simulink model "FCS"  (R2020b)
settings: Solver=VariableStepAuto  StartTime=0.0  StopTime=stabtime+twdw  RelTol=1e-3
undefined symbols (not defined in the file): Capacity, CombinedEDMElectricalPower, CombinedEDMLoss, fuelCellOrg, N, Nom_voltage, OPCircuitDechg, Rincharge, RInDechrg, sigbuilder_block, SOC_initial, SOCR, Time
libraries: powerlib_meascontrol x6, eeStairGenerator x5, simulink x2, powerlib x1
settings Model: Creator=oqz0vm8  LastModifiedBy=dahmani
settings SolverCC: AlgebraicLoopSolver=LineSearch
settings DataIOCC: ReturnWorkspaceOutputs=off
settings DebuggingCC: ArithmeticOperatorsInVariantConditions=warning
settings SFSimCC: SimUseLocalCustomCode=off  CustomCodeUndefinedFunction=UseInterfaceOnly
settings RTWCC: RTWUseLocalCustomCode=off
settings CodeAppCC: StateflowObjectComments=on
settings SimscapeCC: SimscapeNormalizeSystem=off

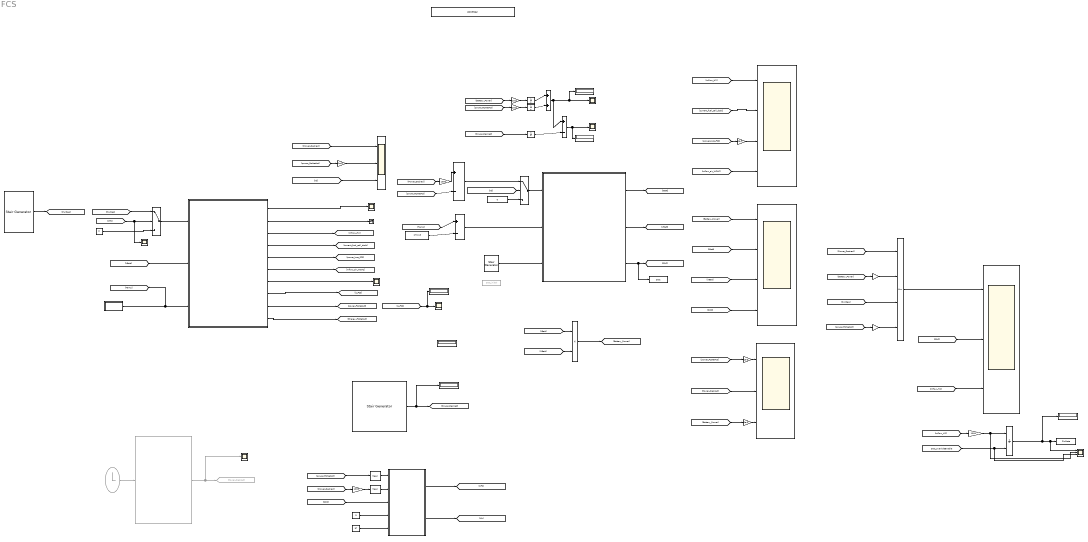
== system FCS ==
  note: Energy balance
  "  " : Gain  Gain=1e-3
  Battery_Model1 : Subsystem
  Clock : Clock  Commented=on
  Combined Drive Motor : Subsystem  Commented=on
  Constant : Constant  Value=273.15
  Constant1 : Constant  Value=0
  Constant4 : Constant  Value=0
  Display{,1..4,6} (6 alike) : Display
  EMS : MATLAB Function  TreatAsAtomicUnit=on
  Gain1 : Gain  Gain=1000
  Gain2 : Gain  Gain=1e-3
  Gain3 : Gain  Gain=1e-3
  Gain4 : Gain  Gain=1000
  Goto : Goto  Commented=on  GotoTag=Power_Desired
  Integrator : Integrator
  Integrator1 : Integrator
  Integrator2 : Integrator
  Integrator3 : Integrator  ExternalReset=either
  "K to °C " : Sum  Inputs=|+-
  "KW to W " : Gain  Gain=1000
  Mean : powerlib_meascontrol/Measurements/Mean  Freq=60  Vinit=1  Ts=0
  Mean1 : powerlib_meascontrol/Measurements/Mean  Freq=60  Vinit=1  Ts=0
  Mux : Mux
  Product : Product
  SOC_initial : eeStairGenerator/Stair Generator  LabelModeActiveChoice=Discrete  TimeInput=SOCInitTime  AmplitudeInput=SOC_overrideValue  SampleTime=1  RepeatPattern=off  OutDataTypeStr=double
      settings: SourceProductBaseCode=PS
  SOC_initial1 : Constant  Commented=on  Value=SOC_initial
  SOCmax : Constant  Value=97
  SOCmin : Constant  Value=3
  Scope : Scope  NumInputPorts=4
  Scope{1..2,5..6,9..10,14} (7 alike) : Scope
  Scope{7..8,11..12} (4 alike) : Scope  NumInputPorts=3
  Scope4 : Scope  NumInputPorts=4
  Stair Generator : eeStairGenerator/Stair Generator  LabelModeActiveChoice=Discrete  TimeInput=FCSimPdesTime  AmplitudeInput=FCSimPdes  SampleTime=1  RepeatPattern=off  OutDataTypeStr=double
      settings: SourceProductBaseCode=PS
  Stair Generator1 : eeStairGenerator/Stair Generator  LabelModeActiveChoice=Discrete  TimeInput=PwrReqTime  AmplitudeInput=PwrReq  SampleTime=1  RepeatPattern=off  OutDataTypeStr=double
      settings: SourceProductBaseCode=PS
  Sum : Sum  Inputs=|+-
  Sum1 : Sum  Inputs=|++
  Sum2 : Sum  Inputs=|+-
  Switch1 : Switch  Criteria=u2 > Threshold
  Switch3 : Switch  Criteria=u2 > Threshold
  Temp(K) : Subsystem  Tag=STV Subsys  LoadFcn=sigbuilder_block('load');  StartFcn=sigbuilder_block('start');  StopFcn=sigbuilder_block('stop');  ClipboardFcn=sigbuilder_block('clipboard');  mask(Sigbuilder block){tuvar=[0:10]}
      mask help: Simulink:masks:SigbuilderBlock_MD
      mask init:
      | if ~strcmp(get_param(bdroot(gcbh),'SimulationStatus'),'stopped') tuvar = sigbuilder_block('maskInit'); end
      settings: CopyFcn=sigbuilder_block('copy');  DeleteFcn=sigbuilder_block('delete');  ModelCloseFcn=sigbuilder_block('modelClose');  PreSaveFcn=sigbuilder_block('preSave');  PauseFcn=sigbuilder_block('pause');  ContinueFcn=sigbuilder_block('continue');  NameChangeFcn=sigbuilder_block('namechange');  OpenFcn=sigbuilder_block('open',[595.8 21.6 550.8 361.2 ]);  CloseFcn=sigbuilder_block('close');
      mask Display: plot(0, 0, 100, 100,[2, 2, 32, 32, 2], [68, 8, 8, 68, 68],[32, 2], [38, 38], [32, 19, 2],[53, 60, 44], [32, 17, 17, 2],[16, 16, 31, 31]);txt = getActiveGroup(gcbh);text(2, 100, txt,'verticalAlignment', 'top');
  Terminator : Terminator
  To Workspace : ToWorkspace  VariableName=FlwRate  SampleTime=-1
      settings: Save2DSignal=2-D array (concatenate along first dimension)
  To Workspace2 : ToWorkspace  VariableName=SOC  SaveFormat=Timeseries  SampleTime=-1
      settings: Save2DSignal=2-D array (concatenate along first dimension)
  W to KW : Gain  Gain=1e-3
  W to KW {1..4} (4 alike) : Gain  Gain=1e-3
  fuelCell_DCDC_Boost_Models : Subsystem
  powergui : powerlib/powergui  Priority=1  SimulationMode=Continuous  SampleTime=50e-6  frequency=60  Iterations=50  frequencyindice=0  Pbase=100e6  ErrMax=1e-4  UnitsV=kV  UnitsW=MW  buscounter=0  FunctionMessages=off  echomessages=off  EnableUseOfTLC=off  CurrentSourceSwitches=off  DisableSnubberDevices=off  DisableRonSwitches=off  DisableVfSwitches=off  DisplayEquations=off  AutomaticDiscreteSolvers=off  SolverType=Tustin/Backward Euler (TBE)  Interpol=off  ExternalGateDelay=off  methode=off  Ts=100  x0status=blocks  SPID=on  SwTol=0  HookPort=off  NonlinearTolerance=1e-4  nMaxIteration=100  ContinueOnMaxIteration=off  RestoreLinks=warning  ResistiveCurrentMeasurement=off  Frange=[0:2:500]  Ylog=off  Xlog=on  ShowGrid=off  save=off  variable=ZData  structure=0  ZoomFFT=off  StartTime=0.0  cycles=1  DisplayStyle=1  fundamental=60  FreqAxis=off  MaxFrequency=1000  frequencyindicesteady=1  RmsSteady=1  display=off
  wires:
  [SOC] -> EMS/3(SOC)
  [Battery_Power] -> Scope/1  "Battery_Power"
  W to KW 4/1 -> Scope4/3  "power_loss_FCS"
  [Kb] -> Switch3/2
  EMS/1(KFC) -> [KFC]
  SOCmin/1 -> EMS/4(SOCmin)
  Temp(K)/1(Signal 1) -> [Temp], fuelCell_DCDC_Boost_Models/3(temp_air_atmo_[K])
  Mean1/1 -> EMS/2(PL)
  Combined Drive Motor/1(Power_Desired_net(KW)) -> Scope2/1, Goto/1
  [Kb] -> Scope8/3
  "KW to W "/1 -> Sum/1
  [VBatt] -> Product/2
  fuelCell_DCDC_Boost_Models/5(power_loss_FCS_[W]) -> [power_loss_FCS]
  [power_loss_FCS] -> W to KW 4/1
  [power_FcsNetAct] -> W to KW 3/1
  Sum/1 -> Switch3/1
  Switch3/1 -> Battery_Model1/1(P_demand(w))
  [power_FcsNetAct] -> Sum/2
  fuelCell_DCDC_Boost_Models/9(power_FcsNetAct) -> [power_FcsNetAct]
  "K to °C "/1 -> Battery_Model1/2(Temp(Cels))
  [Battery_Power] -> W to KW 1/1
  W to KW 3/1 -> Scope8/2  "FuelCell_Power"
  Constant4/1 -> Switch3/3
  [Power_Desired] -> "KW to W "/1
  W to KW 2/1 -> Scope7/1  "FuelCell_Power"
  [Power_Desired] -> Gain1/1
  [Power_Desired] -> Scope7/2  "Power_Desired"
  SOCmax/1 -> EMS/5(SOCmax)
  [Power_Desired] -> Scope8/1  "Power_Desired"
  [mflow_air_WCAC] -> Scope4/4  "mflow_air_WCAC"
  fuelCell_DCDC_Boost_Models/1(info) -> Scope1/1
  fuelCell_DCDC_Boost_Models/2(sensor) -> Terminator/1
  [current_fuel_cell_dcdc] -> Scope4/2  "current_fuel_cell_dcdc"
  [power_FcsNetAct] -> W to KW 2/1
  [mflow_H2] -> Scope4/1  "mflow_H2"
  W to KW 1/1 -> Scope7/3  "Battery_Power"
  EMS/2(Kb) -> [Kb]
  fuelCell_DCDC_Boost_Models/8(U_FCS[V]) -> [U_FCS]
  Gain1/1 -> Mean1/1
  [SOC] -> Scope/4  "SOC"
  [power_FcsNetAct] -> Mean/1
  fuelCell_DCDC_Boost_Models/4(current_fuel_cell_dcdc_[A]) -> [current_fuel_cell_dcdc]
  Mean/1 -> EMS/1(PFC)
  fuelCell_DCDC_Boost_Models/6(mflow_air_WCAC_[kg.s-1]) -> [mflow_air_WCAC]
  [IBatt] -> Product/1
  [IBatt] -> Scope/2  "Battery_current"
  Battery_Model1/3(.SOC) -> To Workspace2/1, [SOC]
  Clock/1 -> Combined Drive Motor/1(Time(s))
  [U_FCS] -> Display2/1, Scope5/1
  Constant/1 -> "K to °C "/2
  Battery_Model1/2(.VBatt) -> [VBatt]
  [VBatt] -> Scope/3  "Battery_voltage"
  Battery_Model1/1(Ibat) -> [IBatt]
  fuelCell_DCDC_Boost_Models/7(power_StackAct_[W]) -> Scope6/1
  [Temp] -> "K to °C "/1
  Sum2/1 -> Scope10/1, Display/1
  Sum1/1 -> Display1/1, Scope14/1, Sum2/1
  [Battery_Power] -> "  "/1
  Integrator/1 -> Sum1/2
  Integrator2/1 -> Sum2/2
  W to KW/1 -> Integrator/1
  Integrator1/1 -> Sum1/1
  [power_FcsNetAct] -> W to KW/1
  [Power_Desired] -> Integrator2/1
  "  "/1 -> Integrator1/1
  [VBatt] -> fuelCell_DCDC_Boost_Models/2(voltage_out_epsBattTracOrg_[V])
  SOC_initial/1 -> Battery_Model1/3(SOC_initial)
  Stair Generator/1 -> Display4/1, [Power_Desired]
  fuelCell_DCDC_Boost_Models/3(mflow_H2_[kg.s-1]) -> [mflow_H2]
  Constant1/1 -> Switch1/3
  [PwrReq] -> Switch1/1
  [KFC] -> Scope9/1, Switch1/2
  Switch1/1 -> fuelCell_DCDC_Boost_Models/1(FcsPwrReq(Kw))
  Stair Generator1/1 -> [PwrReq]
  [Power_Desired] -> Mux/1  "Power_Desired"
  Mux/1 -> Scope12/1
  [Battery_Power] -> Gain2/1
  Gain2/1 -> Mux/2  "Battery_Power"
  [PwrReq] -> Mux/3  "PwrReq"
  [power_FcsNetAct] -> Gain3/1
  Gain3/1 -> Mux/4  "power_FcsNetAct"
  [SOC] -> Scope12/2  "SOC"
  [mflow_H2] -> Scope12/3  "mflow_H2"
  [SOC_overrideEnable] -> Scope11/3, Integrator3/2  "SOC_overrideEnable"
  Integrator3/1 -> Display6/1, Scope11/1, To Workspace/1
  [mflow_H2] -> Gain4/1
  Gain4/1 -> Scope11/2, Integrator3/1
  fuelCell_DCDC_Boost_Models/10(Energy_FcsNetAct) -> [Energy_FcsNetAct]
  Product/1 -> [Battery_Power]

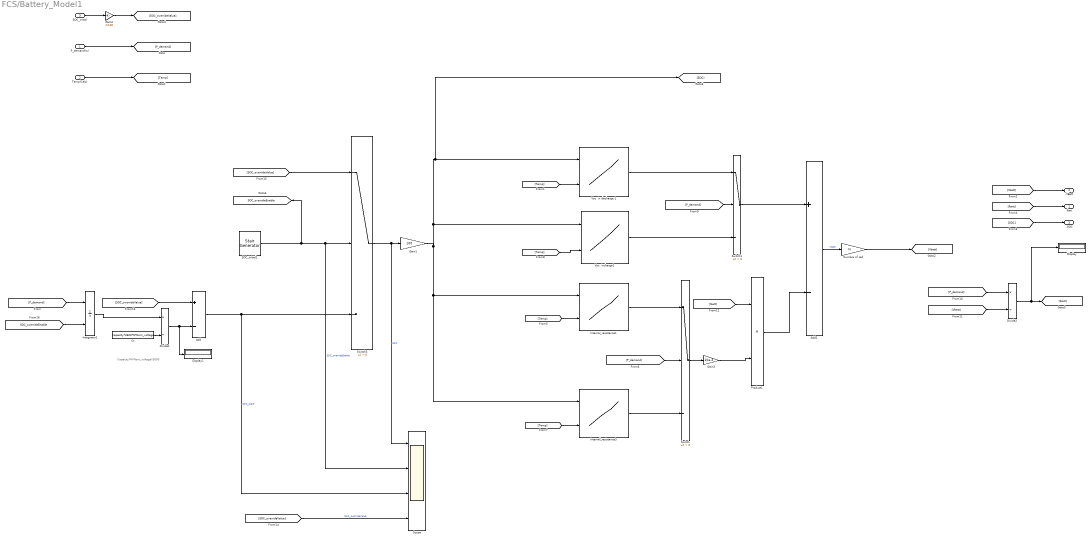
== system FCS/Battery_Model1 ==
  note: Capacity*N*Nom_voltage*3600
  P_demand(w) : Inport
  Temp(Cels) : Inport  Port=2
  SOC_initial : Inport  Port=3
  Add : Sum  Inputs=+-
  Add2 : Sum  Inputs=+-
  "Ct " : Constant  Value=Capacity*3600*N*Nom_voltage
  Display : Display
  Display1 : Display
  Divide1 : Product  Inputs=*/
  Divide2 : Product  Inputs=*/
  Gain1 : Gain  Gain=100
  Gain2 : Gain  Gain=1/100
  Gain3 : Gain  Gain=10e-3
  Integrator2 : Integrator  ExternalReset=either
  Internal_resistance1 : Lookup_n-D  BreakpointsForDimension1=SOCR  BreakpointsForDimension2=|  BreakpointsForDimension3=[5, 7]  Table=RInDechrg  InternalRulePriority=Speed  RndMeth=Simplest  InputSameDT=on
      | [-20 -10 0 5 10 20 25 35 45 50
      | ]
      settings: InputPortMap=u0,u1
  Internal_resistance3 : Lookup_n-D  BreakpointsForDimension1=|  BreakpointsForDimension2=|  BreakpointsForDimension3=[5, 7]  Table=Rincharge  InternalRulePriority=Speed  RndMeth=Simplest  InputSameDT=on
      BreakpointsForDimension1=|
      | [3
      | ;5
      | ;10
      | ;15
      | ;20
      | ;25
      | ;30
      | ;35
      | ;40
      | ;45
      | ;50
      | ;55
      | ;60
      | ;65
      | ;70
      | ;75
      | ;80
      | ;85
      | ;90
      | ;95
      | ;97]
      BreakpointsForDimension2=|
      | [-20 -10 0 5 10 20 25 35 45 50
      | ]
      settings: InputPortMap=u0,u1
  Numbre of cell : Gain  Gain=N
  Product1 : Product
  SOC_initial2 : eeStairGenerator/Stair Generator  LabelModeActiveChoice=Discrete  TimeInput=SOCInitTime  AmplitudeInput=SOC_overrideEnable  SampleTime=1  RepeatPattern=off  OutDataTypeStr=double
      settings: SourceProductBaseCode=PS
  Scope : Scope  NumInputPorts=4
  Switch : Switch  Criteria=u2 > Threshold
  Switch1 : Switch  Criteria=u2 > Threshold
  Switch3 : Switch  Criteria=u2 > Threshold
  Voc  in decharge 1 : Lookup_n-D  BreakpointsForDimension1=|  BreakpointsForDimension2=|  BreakpointsForDimension3=[5, 7]  Table=OPCircuitDechg  InternalRulePriority=Speed  RndMeth=Simplest  InputSameDT=on
      BreakpointsForDimension1=|
      | [0;
      | 3
      | ;5
      | ;10
      | ;15
      | ;20
      | ;25
      | ;30
      | ;35
      | ;40
      | ;45
      | ;50
      | ;55
      | ;60
      | ;65
      | ;70
      | ;75
      | ;80
      | ;85
      | ;90
      | ;95
      | ;97;
      | 100]
      BreakpointsForDimension2=|
      | [-20 -10 0 5 10 20 25 35 45 50
      | ]
      settings: InputPortMap=u0,u1
  Voc  incharge1 : Lookup_n-D  BreakpointsForDimension1=|  BreakpointsForDimension2=|  BreakpointsForDimension3=[5, 7]  Table=|  InternalRulePriority=Speed  RndMeth=Simplest  InputSameDT=on
      BreakpointsForDimension1=|
      | [0;
      | 3
      | ;5
      | ;10
      | ;15
      | ;20
      | ;25
      | ;30
      | ;35
      | ;40
      | ;45
      | ;50
      | ;55
      | ;60
      | ;65
      | ;70
      | ;75
      | ;80
      | ;85
      | ;90
      | ;95
      | ;97;
      | 100]
      Table=|
      | [3.004	3.004	3.004	3.004	3.004	2.998	2.995	2.984	2.973	2.967
      | ;3.191	3.191	3.191	3.191	3.191	3.097	3.186	3.174	3.163	3.157
      | ;3.316	3.316	3.316	3.316	3.316	3.163	3.313	3.301	3.289	3.283
      | ;3.414	3.414	3.414	3.414	3.414	3.263	3.412	3.397	3.381	3.374
      | ;3.461	3.461	3.461	3.461	3.461	3.385	3.461	3.459	3.458	3.457
      | ;3.510	3.510	3.510	3.510	3.510	3.468	3.511	3.506	3.502	3.500
      | ;3.561	3.561	3.561	3.561	3.561	3.505	3.562	3.556	3.550	3.548
      | ;3.602	3.602	3.602	3.602	3.602	3.559	3.603	3.599	3.596	3.594
      | ;3.629	3.629	3.629	3.629	3.629	3.603	3.630	3.631	3.633	3.633
      | ;3.655	3.655	3.655	3.655	3.655	3.643	3.657	3.662	3.668	3.671
      | ;3.688	3.688	3.688	3.688	3.688	3.677	3.690	3.696	3.703	3.706
      | ;3.732	3.732	3.732	3.732	3.732	3.721	3.735	3.740	3.746	3.749
      | ;3.788	3.788	3.788	3.788	3.788	3.773	3.790	3.792	3.795	3.796
      | ;3.852	3.852	3.852	3.852	3.852	3.827	3.854	3.849	3.844	3.842
      | ;3.899	3.899	3.899	3.899	3.899	3.892	3.900	3.895	3.890	3.887
      | ;3.938	3.938	3.938	3.938	3.938	3.932	3.939	3.938	3.938	3.938
      | ;3.986	3.986	3.986	3.986	3.986	3.982	3.987	3.986	3.985	3.984
      | ;4.044	4.044	4.044	4.044	4.044	4.041	4.045	4.041	4.038	4.037
      | ;4.090	4.090	4.090	4.090	4.090	4.086	4.091	4.086	4.082	4.080
      | ;4.107	4.107	4.107	4.107	4.107	4.103	4.109	4.105	4.102	4.100
      | ;4.123	4.123	4.123	4.123	4.123	4.121	4.125	4.121	4.118	4.117
      | ;4.136	4.136	4.136	4.136	4.136	4.140	4.138	4.134	4.131	4.129
      | ;4.157	4.157	4.157	4.157	4.157	4.169	4.159	4.154	4.149	4.147
      | ]
      BreakpointsForDimension2=|
      | [-20 -10 0 5 10 20 25 35 45 50
      | ]
      settings: InputPortMap=u0,u1
  Ibat : Outport
  .VBatt : Outport  Port=2
  .SOC : Outport  Port=3
  tag scope: SOC_overrideEnable=global
  wires:
  [Ibatt] -> Product1/1
  Divide2/1 -> [Ibatt], Display/1
  Switch1/1 -> Add2/1
  [P_demand] -> Switch1/2
  Voc  in decharge 1/1 -> Switch1/1
  Voc  incharge1/1 -> Switch1/3
  [Temp] -> Voc  incharge1/2
  [Temp] -> Internal_resistance3/2
  [P_demand] -> Switch/2
  Internal_resistance3/1 -> Switch/3
  Internal_resistance1/1 -> Switch/1
  Switch/1 -> Gain3/1
  [Temp] -> Internal_resistance1/2
  Gain3/1 -> Product1/2
  [Vbatt] -> .VBatt/1
  [Ibatt] -> Ibat/1
  [SOC] -> .SOC/1
  Temp(Cels)/1 -> [Temp]
  P_demand(w)/1 -> [P_demand]
  [Temp] -> Voc  in decharge 1/2
  Integrator2/1 -> Divide1/1
  Product1/1 -> Add2/2
  Add2/1 -> Numbre of cell/1  "Vbatt"
  [P_demand] -> Integrator2/1
  Divide1/1 -> Display1/1, Add/2
  [SOC_overrideValue] -> Switch3/1
  Add/1 -> Switch3/3, Scope/3  "SOC_plant"
  SOC_initial2/1 -> [SOC_overrideEnable], Scope/2, Switch3/2  "SOC_overrideEnable"
  "Ct "/1 -> Divide1/2
  [SOC_overrideValue] -> Add/1
  Gain1/1 -> Internal_resistance3/1, Internal_resistance1/1, Voc  incharge1/1, [SOC], Voc  in decharge 1/1
  Switch3/1 -> Scope/1, Gain1/1  "SOC"
  SOC_initial/1 -> Gain2/1
  Gain2/1 -> [SOC_overrideValue]
  [SOC_overrideValue] -> Scope/4  "SOC_overrideValue"
  [SOC_overrideEnable] -> Integrator2/2
  [Vbatt] -> Divide2/2
  Numbre of cell/1 -> [Vbatt]
  [P_demand] -> Divide2/1

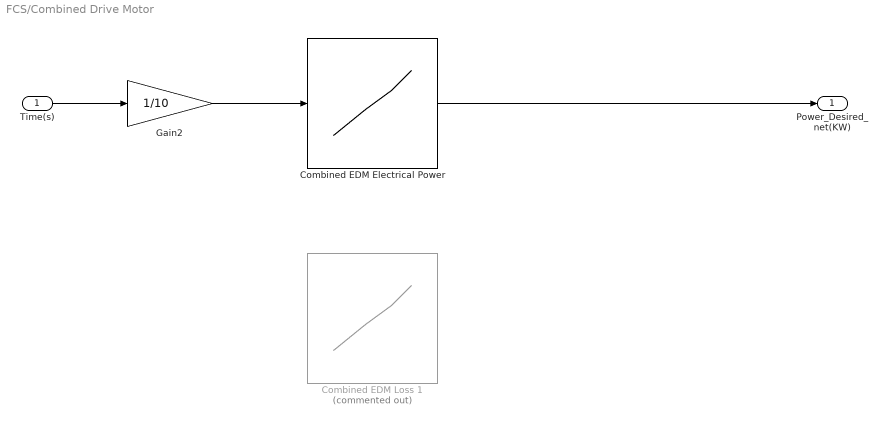
== system FCS/Combined Drive Motor ==
  Time(s) : Inport
  Combined EDM Electrical Power : Lookup_n-D  NumberOfTableDimensions=1  LookupTableObject=''  BreakpointsForDimension1=Time  BreakpointsForDimension1FirstPoint=10  BreakpointsForDimension2FirstPoint=10  BreakpointsForDimension1Spacing=12  BreakpointsForDimension2Spacing=12  Table=CombinedEDMElectricalPower  InternalRulePriority=Speed  RndMeth=Simplest  InputSameDT=on
  Combined EDM Loss 1 : Lookup_n-D  Commented=on  NumberOfTableDimensions=1  LookupTableObject=''  BreakpointsForDimension1=Time  BreakpointsForDimension1FirstPoint=10  BreakpointsForDimension2FirstPoint=10  BreakpointsForDimension1Spacing=12  BreakpointsForDimension2Spacing=12  Table=CombinedEDMLoss  InternalRulePriority=Speed  RndMeth=Simplest  InputSameDT=on
  Gain2 : Gain  Gain=1/10
  Power_Desired_net(KW) : Outport
  wires:
  Combined EDM Electrical Power/1 -> Power_Desired_net(KW)/1
  Time(s)/1 -> Gain2/1
  Gain2/1 -> Combined EDM Electrical Power/1

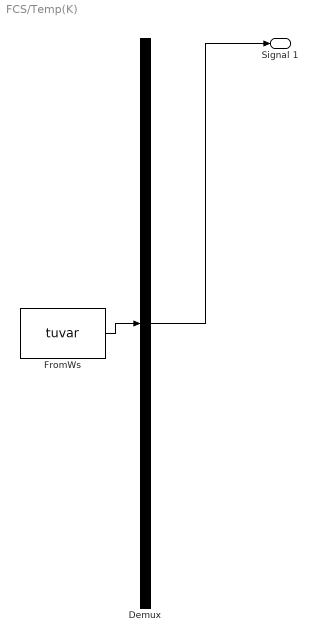
== system FCS/Temp(K) ==
  Demux : Demux  Tag=STV Demux  Outputs=1
      settings: DisplayOption=none
  FromWs : FromWorkspace  Tag=STV FromWs  VariableName=tuvar
      SigBuilderData=|
      | common.afterFinalStr = 'Extrapolate'
      | common.sampleTime = 0
      | dataSet.timeRange = [0 10]
      | dataSet.name = 'Group 1'
      | sbobj.Groups.Name = 'Group 1'
      | sbobj.Groups.Signals.Name = 'Signal 1'
      | sbobj.Groups.Signals.XData = [0 4 4 6 6 10]
      | sbobj.Groups.Signals.YData = [290 290 293 293 295 295]
  Signal 1 : Outport  Tag=STV Outport
  wires:
  Demux/1 -> Signal 1/1
  FromWs/1 -> Demux/1

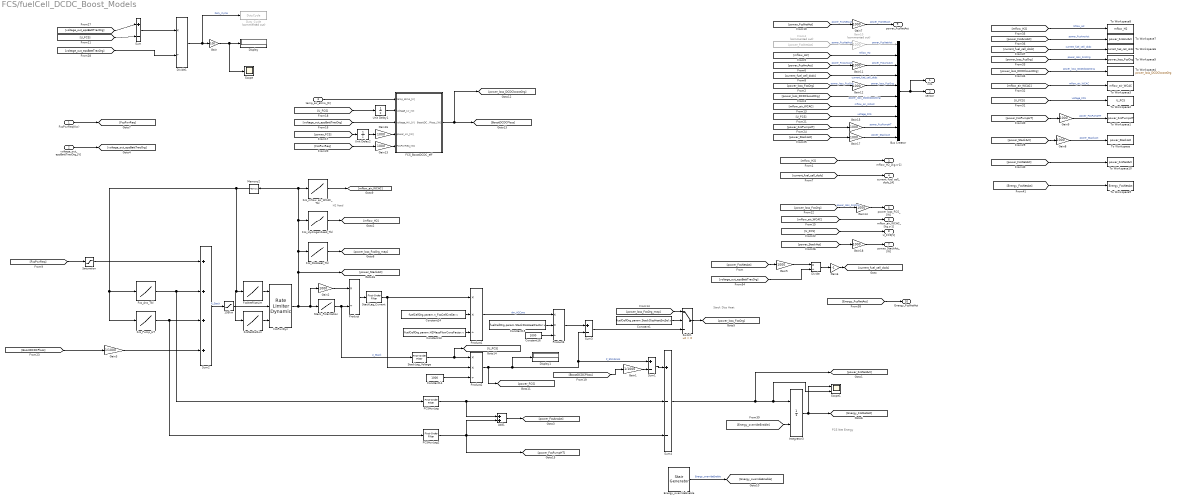
== system FCS/fuelCell_DCDC_Boost_Models ==
  note: FCS Net Energy
  note: Stack Diss Heat
  note: H2 feed
  FcsPwrReq(Kw) : Inport
  voltage_out_epsBattTracOrg_[V] : Inport  Port=2
  temp_air_atmo_[K] : Inport  Port=3
  195kw : Saturate  UpperLimit=max(fuelCellOrg.param.Fcs_Anc_Tbl.x)  LowerLimit=0
  Add1 : Sum
  Bus Creator : BusCreator  Inputs=10
  Constant1 : Constant  Value=fuelCellOrg.param.StackDissHeatSrcSel.v
  Constant13 : Constant  Value=fuelCellOrg.param.H2MassFlowConsFactor.v
  Constant14 : Constant  Value=1000
  Constant15 : Constant  Value=fuelCellOrg.param.StackDissHeatFactor.v
  Constant16 : Constant  Value=1000
  Constant24 : Constant  Value=fuelCellOrg.param.n_FcsCellCntSer.v
  Display : Display
  Display1 : Display
  Divide : Product  Inputs=*/
  Divide1 : Product  Inputs=*/
  Duty_Cycle : ToWorkspace  Commented=on  VariableName=DutyCycle  SaveFormat=Timeseries  SampleTime=-1
  Energy_overrideEnable : eeStairGenerator/Stair Generator  LabelModeActiveChoice=Discrete  TimeInput=Enery_Time  AmplitudeInput=Energy_overrideEnable  SampleTime=1  RepeatPattern=off  OutDataTypeStr=double
      settings: SourceProductBaseCode=PS
  FCSAuxLag : powerlib_meascontrol/Filters/First-Order Filter  FilterType=Lowpass  Tc=fuelCellOrg.param.t_FcsAncLag.v  Ts=0  Initialize=on  Vac_Init=[0, 0, 60]  Vdc_Init=0  PlotResponse=off  FreqRange="[0,  200,  1]"
  FCSAuxLag2 : powerlib_meascontrol/Filters/First-Order Filter  FilterType=Lowpass  Tc=fuelCellOrg.param.t_FcsAncLag.v  Ts=0  Initialize=on  Vac_Init=[0, 0, 60]  Vdc_Init=0  PlotResponse=off  FreqRange="[0,  200,  1]"
  FCS_BoostDCDC_eff : Subsystem
  FcsNetFallLim : Lookup_n-D  NumberOfTableDimensions=1  BreakpointsForDimension1=fuelCellOrg.param.FcsNetFallLim.x  Table=fuelCellOrg.param.FcsNetFallLim.v  ExtrapMethod=Clip  UseLastTableValue=on  InternalRulePriority=Speed  RndMeth=Simplest  InputSameDT=on
  FcsNetRiseLim : Lookup_n-D  NumberOfTableDimensions=1  BreakpointsForDimension1=fuelCellOrg.param.FcsNetRiseLim.x  Table=fuelCellOrg.param.FcsNetRiseLim.v  ExtrapMethod=Clip  UseLastTableValue=on  InternalRulePriority=Speed  RndMeth=Simplest  InputSameDT=on
  FcsPwrDyn : simulink/Discontinuities/Rate Limiter Dynamic
  Fcs_Anc_Tbl : Lookup_n-D  NumberOfTableDimensions=1  BreakpointsForDimension1=fuelCellOrg.param.Fcs_Anc_Tbl.x  Table=fuelCellOrg.param.Fcs_Anc_Tbl.v  ExtrapMethod=Clip  UseLastTableValue=on  InternalRulePriority=Speed  RndMeth=Simplest  InputSameDT=on
  Fcs_DissHeat_Tbl : Lookup_n-D  NumberOfTableDimensions=1  BreakpointsForDimension1=fuelCellOrg.param.Fcs_DissHeat_Tbl.x  Table=fuelCellOrg.param.Fcs_DissHeat_Tbl.v  ExtrapMethod=Clip  UseLastTableValue=on  InternalRulePriority=Speed  RndMeth=Simplest  InputSameDT=on
  Fcs_HydrogenFeed_Tbl : Lookup_n-D  NumberOfTableDimensions=1  BreakpointsForDimension1=fuelCellOrg.param.Fcs_HydrogenFeed_Tbl.x  Table=fuelCellOrg.param.Fcs_HydrogenFeed_Tbl.v  ExtrapMethod=Clip  UseLastTableValue=on  InternalRulePriority=Speed  RndMeth=Simplest  InputSameDT=on
  Fcs_Pump_HT : Lookup_n-D  NumberOfTableDimensions=1  BreakpointsForDimension1=fuelCellOrg.param.P_FcsPumpHT.x  Table=fuelCellOrg.param.P_FcsPumpHT.v  ExtrapMethod=Clip  UseLastTableValue=on  InternalRulePriority=Speed  RndMeth=Simplest  InputSameDT=on
  Fcs_mflow_air_WCAC_Tbl : Lookup_n-D  NumberOfTableDimensions=1  BreakpointsForDimension1=fuelCellOrg.param.Fcs_mflow_air_WCAC_Tbl.x  Table=fuelCellOrg.param.Fcs_mflow_air_WCAC_Tbl.v  ExtrapMethod=Clip  UseLastTableValue=on  InternalRulePriority=Speed  RndMeth=Simplest  InputSameDT=on
  From4 : From  Commented=on  GotoTag=power_FcsNetAct
  Gain : Gain  Gain=100
  Gain1 : Gain  Gain=1/1000
  Gain10 : Gain  Commented=on  Gain=1000
  Gain{2,5,7..9,11..18} (13 alike) : Gain  Gain=1000
  Gain3 : Gain  Gain=1/1000
  Gain6 : Gain  Gain=-1
  Integrator3 : Integrator  ExternalReset=either
  Memory2 : Memory
  Product : Product  Inputs=*/
  Product1 : Product  Inputs=**/
  Product2 : Product  Inputs=**/
  Product3 : Product  Inputs=**/
  Saturation : Saturate  UpperLimit=fuelCellOrg.param.P_FcsNetMaxLim.v  LowerLimit=0
  Scope : Scope
  Scope1 : Scope  NumInputPorts=2
  StackLag_Current : powerlib_meascontrol/Filters/First-Order Filter  FilterType=Lowpass  Tc=fuelCellOrg.param.t_StckCurrLag.v  Ts=0  Initialize=on  Vac_Init=[0, 0, 60]  Vdc_Init=0  PlotResponse=off  FreqRange="[0,  200,  1]"
  StackLag_Voltage : powerlib_meascontrol/Filters/First-Order Filter  FilterType=Lowpass  Tc=fuelCellOrg.param.t_StckVoltLag.v  Ts=0  Initialize=on  Vac_Init=[0, 0, 60]  Vdc_Init=0  PlotResponse=off  FreqRange="[0,  200,  1]"
  Stack_Polarization : Lookup  InputValues=fuelCellOrg.param.StackPolarization.x  Table=fuelCellOrg.param.StackPolarization.v  LookUpMeth=Interpolation-Use End Values
  Sum : Sum  Inputs=|+-
  Sum1 : Sum  Inputs=+-
  Sum2 : Sum  Inputs=++++
  Sum3 : Sum  Inputs=+-
  Sum4 : Sum  Inputs=+--
  Switch : Switch  Criteria=u2 > Threshold
  To Workspace : ToWorkspace  VariableName=power_StackAct  SaveFormat=Timeseries  SampleTime=-1
  To Workspace1 : ToWorkspace  VariableName=power_FcsPumpHT  SaveFormat=Timeseries  SampleTime=-1
  To Workspace10 : ToWorkspace  VariableName=power_FcsNetAct  SaveFormat=Timeseries  SampleTime=-1
  To Workspace2 : ToWorkspace  VariableName=U_FCS  SaveFormat=Timeseries  SampleTime=-1
  To Workspace3 : ToWorkspace  VariableName=mflow_air_WCAC  SaveFormat=Timeseries  SampleTime=-1
  To Workspace4 : ToWorkspace  VariableName=power_loss_DCDCboostOrg  SaveFormat=Timeseries  SampleTime=-1
  To Workspace5 : ToWorkspace  VariableName=power_loss_FcsOrg  SaveFormat=Timeseries  SampleTime=-1
  To Workspace6 : ToWorkspace  VariableName=current_fuel_cell_dcdc  SaveFormat=Timeseries  SampleTime=-1
  To Workspace7 : ToWorkspace  VariableName=power_FcsAncAct  SaveFormat=Timeseries  SampleTime=-1
  To Workspace8 : ToWorkspace  VariableName=mflow_H2  SaveFormat=Timeseries  SampleTime=-1
  To Workspace9 : ToWorkspace  VariableName=Energy_FcsNetAct  SampleTime=-1
      settings: Save2DSignal=2-D array (concatenate along first dimension)
  Unit Delay1 : UnitDelay  SampleTime=-1  HasFrameUpgradeWarning=on
  Unit Delay2 : UnitDelay  SampleTime=-1  HasFrameUpgradeWarning=on
  info : Outport
  sensor : Outport  Port=2
  mflow_H2_[kg.s-1] : Outport  Port=3
  current_fuel_cell_dcdc_[A] : Outport  Port=4
  power_loss_FCS_[W] : Outport  Port=5
  mflow_air_WCAC_[kg.s-1] : Outport  Port=6
  power_StackAct_[W] : Outport  Port=7
  U_FCS[V] : Outport  Port=8
  power_FcsNetAct : Outport  Port=9
  Energy_FcsNetAct : Outport  Port=10
  wires:
  195kw/1 -> FcsPwrDyn/2
  Fcs_Pump_HT/1 -> Sum2/3, FCSAuxLag2/1
  FCSAuxLag2/1 -> Sum4/3, Add1/2, [power_FcsPumpHT]
  Constant15/1 -> Product3/2
  Add1/1 -> [power_FcsAncAct]
  Gain3/1 -> Sum2/4
  [mflow_H2] -> mflow_H2_[kg.s-1]/1
  Gain17/1 -> Bus Creator/10  "power_StackAct"
  Gain18/1 -> power_StackAct_[W]/1
  Fcs_DissHeat_Tbl/1 -> [power_loss_FcsOrg_map]
  Gain1/1 -> Sum1/2
  FcsNetFallLim/1 -> FcsPwrDyn/3
  Gain15/1 -> Bus Creator/9  "power_FcsPumpHT"
  Fcs_mflow_air_WCAC_Tbl/1 -> [mflow_air_WCAC]
  FcsNetRiseLim/1 -> FcsPwrDyn/1
  Product3/1 -> Sum3/1
  FcsPwrDyn/1 -> Stack_Polarization/1, Gain2/1, [power_StackAct], Fcs_HydrogenFeed_Tbl/1, Memory2/1, Fcs_mflow_air_WCAC_Tbl/1, Fcs_DissHeat_Tbl/1
  Switch/1 -> [power_loss_FcsOrg]
  Gain13/1 -> FCS_BoostDCDC_eff/5(FcsPwrReq_[W])
  [BoostDCDCPloss] -> Gain3/1
  [mflow_air_WCAC] -> mflow_air_WCAC_[kg.s-1]/1
  Product1/1 -> Product3/1  "dm_H2Cons"
  Constant24/1 -> Product1/2
  StackLag_Voltage/1 -> Product2/1, [U_FCS]
  Constant13/1 -> Product1/3
  [power_StackAct] -> Gain17/1
  Bus Creator/1 -> sensor/1, info/1
  From4/1 -> Gain10/1  "power_FcsNetAct"
  [BoostDCDCPloss] -> Gain1/1
  [power_loss_FcsOrg_map] -> Switch/1
  Saturation/1 -> Sum2/1
  Product2/1 -> [power_FCS], Display1/1, Sum3/2, Sum1/1  "P_StckGross"
  Fcs_HydrogenFeed_Tbl/1 -> [mflow_H2]
  Constant14/1 -> Product2/3
  StackLag_Current/1 -> Product1/1, Product2/2
  Constant1/1 -> Switch/2
  Sum2/1 -> 195kw/1  "P_Stack"
  [power_StackAct] -> Gain18/1
  [mflow_air_WCAC] -> Bus Creator/7  "mflow_air_WCAC"
  [FcsPwrReq] -> Gain13/1
  [power_FcsPumpHT] -> Gain15/1
  Integrator3/1 -> [Energy_FcsNetAct], Scope1/1
  [U_FCS] -> Bus Creator/8  "voltage_FCS"
  FCSAuxLag/1 -> Sum4/2, Add1/1
  [FcsPwrReq] -> Saturation/1
  Product/1 -> StackLag_Current/1
  Gain2/1 -> Product/1
  Sum1/1 -> Sum4/1
  Constant16/1 -> Product3/3
  Stack_Polarization/1 -> StackLag_Voltage/1, Product/2  "U_Stack"
  [power_FcsAncAct] -> Gain11/1  "power_FcsAncAct"
  [U_FCS] -> Unit Delay1/1
  [power_loss_DCDCboostOrg] -> Bus Creator/6  "power_loss_DCDCboostOrg"
  Divide/1 -> Gain6/1
  [current_fuel_cell_dcdc] -> current_fuel_cell_dcdc_[A]/1
  [voltage_out_epsBattTracOrg] -> FCS_BoostDCDC_eff/3(voltage_HV_[V])
  Unit Delay2/1 -> Gain16/1
  [power_FCS] -> Unit Delay2/1
  [mflow_H2] -> Bus Creator/2  "mflow_H2"
  Gain5/1 -> Divide/1
  Sum3/1 -> Switch/3
  FCS_BoostDCDC_eff/1(BoostDCDCPloss_[W]) -> [BoostDCDCPloss], [power_loss_DCDCboostOrg]
  Gain6/1 -> [current_fuel_cell_dcdc]
  Gain10/1 -> Bus Creator/1  "power_FcsNetAct"
  Gain16/1 -> FCS_BoostDCDC_eff/4(power_LV_[W])
  voltage_out_epsBattTracOrg_[V]/1 -> [voltage_out_epsBattTracOrg]
  [power_FcsNetAct] -> Gain5/1
  Fcs_Anc_Tbl/1 -> FCSAuxLag/1, Sum2/2
  Gain11/1 -> Bus Creator/3  "power_FcsAncAct"
  Gain14/1 -> power_loss_FCS_[W]/1
  [voltage_out_epsBattTracOrg] -> Divide/2
  Gain12/1 -> Bus Creator/5  "power_loss_FcsOrg"
  [current_fuel_cell_dcdc] -> Bus Creator/4  "current_fuel_cell_dcdc"
  Unit Delay1/1 -> FCS_BoostDCDC_eff/2(voltage_LV_[V])
  temp_air_atmo_[K]/1 -> FCS_BoostDCDC_eff/1(temp_atmo_[K])
  [power_loss_FcsOrg] -> Gain12/1  "power_loss_FcsOrg"
  FcsPwrReq(Kw)/1 -> [FcsPwrReq]
  [power_loss_FcsOrg] -> Gain14/1  "power_loss_FcsOrg"
  [U_FCS] -> U_FCS[V]/1
  [power_FcsNetAct] -> Gain7/1  "power_FcsNetAct"
  Gain7/1 -> power_FcsNetAct/1  "power_FcsNetAct"
  [U_FCS] -> Sum/2
  [voltage_out_epsBattTracOrg] -> Sum/1
  Sum/1 -> Divide1/1
  [voltage_out_epsBattTracOrg] -> Divide1/2
  Divide1/1 -> Duty_Cycle/1, Gain/1  "Duty_Cycle"
  [power_StackAct] -> Gain8/1
  Gain8/1 -> To Workspace/1  "power_StackAct"
  [power_FcsPumpHT] -> Gain9/1
  Gain9/1 -> To Workspace1/1  "power_FcsPumpHT"
  [U_FCS] -> To Workspace2/1  "voltage_FCS"
  [mflow_air_WCAC] -> To Workspace3/1  "mflow_air_WCAC"
  [mflow_H2] -> To Workspace8/1  "mflow_H2"
  [power_FcsAncAct] -> To Workspace7/1  "power_FcsAncAct"
  [current_fuel_cell_dcdc] -> To Workspace6/1  "current_fuel_cell_dcdc"
  [power_loss_FcsOrg] -> To Workspace5/1  "power_loss_FcsOrg"
  [power_loss_DCDCboostOrg] -> To Workspace4/1  "power_loss_DCDCboostOrg"
  Gain/1 -> Display/1, Scope/1
  [Energy_FcsNetAct] -> Energy_FcsNetAct/1
  Sum4/1 -> Scope1/2, Integrator3/1, [power_FcsNetAct]
  [Energy_overrideEnable] -> Integrator3/2
  Memory2/1 -> FcsNetFallLim/1, FcsNetRiseLim/1, Fcs_Pump_HT/1, Fcs_Anc_Tbl/1
  Energy_overrideEnable/1 -> [Energy_overrideEnable]  "Energy_overrideEnable"
  [power_FcsNetAct] -> To Workspace10/1
  [Energy_FcsNetAct] -> To Workspace9/1

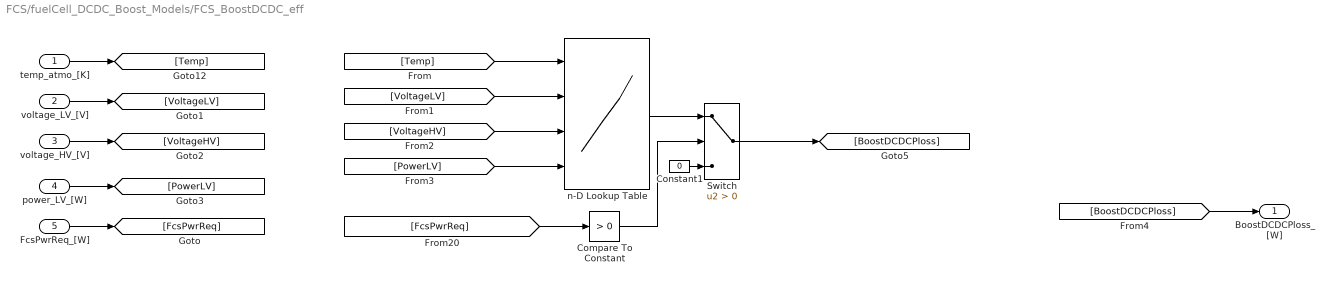
== system FCS/fuelCell_DCDC_Boost_Models/FCS_BoostDCDC_eff ==
  temp_atmo_[K] : Inport
  voltage_LV_[V] : Inport  Port=2
  voltage_HV_[V] : Inport  Port=3
  power_LV_[W] : Inport  Port=4
  FcsPwrReq_[W] : Inport  Port=5
  Compare To Constant : simulink/Logic and Bit Operations/Compare To Constant  relop=>  const=0  OutDataTypeStr=boolean
  Constant1 : Constant  Value=0
  Switch : Switch  Criteria=u2 > Threshold
  n-D Lookup Table : Lookup_n-D  NumberOfTableDimensions=4  BreakpointsForDimension1=fuelCellOrg.param.eta_DcDcBoostMap4d.Temp  BreakpointsForDimension2=fuelCellOrg.param.eta_DcDcBoostMap4d.VoltageLV  BreakpointsForDimension3=fuelCellOrg.param.eta_DcDcBoostMap4d.VoltageHV  BreakpointsForDimension4=fuelCellOrg.param.eta_DcDcBoostMap4d.PowerLV  Table=fuelCellOrg.param.eta_DcDcBoostMap4d.v  InternalRulePriority=Speed  RndMeth=Simplest  InputSameDT=on
      settings: InputPortMap=u0,u1,u2,u3
  BoostDCDCPloss_[W] : Outport
  wires:
  FcsPwrReq_[W]/1 -> [FcsPwrReq]
  [FcsPwrReq] -> Compare To Constant/1
  Switch/1 -> [BoostDCDCPloss]
  [BoostDCDCPloss] -> BoostDCDCPloss_[W]/1
  [VoltageLV] -> n-D Lookup Table/2
  [Temp] -> n-D Lookup Table/1
  power_LV_[W]/1 -> [PowerLV]
  voltage_HV_[V]/1 -> [VoltageHV]
  voltage_LV_[V]/1 -> [VoltageLV]
  temp_atmo_[K]/1 -> [Temp]
  n-D Lookup Table/1 -> Switch/1
  [VoltageHV] -> n-D Lookup Table/3
  Constant1/1 -> Switch/3
  Compare To Constant/1 -> Switch/2
  [PowerLV] -> n-D Lookup Table/4

== matlab function FCS/EMS ==
  data: PFC input; KFC output; PL input; Kb output; SOC input; SOCmin input; SOCmax input

function [KFC,Kb]  = State(PFC, PL ,SOC,SOCmin, SOCmax) 
dataType = 'double';
Pi=PFC-PL;
if PL>0  
    if Pi > 0
        if SOC < SOCmax
            KFC =1;
            Kb =1;
            
        else 
            KFC =1;
            Kb =0;
        end
     else
        if SOC > SOCmin
            if PFC == 0
               KFC =0;
               Kb =1;    
            else
               KFC =1;
               Kb =1;
            end
        else
               KFC =0;
               Kb =0;  
        end
    end
else 
    if SOC > SOCmin && SOC < SOCmax
        KFC =0;
        Kb =1;
    else
               KFC =0;
               Kb =0;  
    end
end
